simulink model "AcasXuClosedLoop_m_1"  (R2019b)
settings: Solver=VariableStepAuto  StartTime=0.0  StopTime=30  RelTol=1e-3
libraries: neural x1560, simulink x2
(part 4 of 85)

== system AcasXuClosedLoop_m_1/networks/AcasXu_4_1/Layer 3 ==
  "a{2} " : Inport  PortDimensions=50
      mask Display: e = 0.06;c1 = [120 230 180]/255;c2 = ([120 230 180]+0)/(256+128);c3 = ([120 230 180]+128)/(256+128);patch([0 1 1 0],[0 0 1 1],c1);patch([0 1 1 1-e 1-e 0+e],[0 0 1 1-e 0+e 0+e],c2);patch([0 0 1 1-e 0+e 0+e],[0 1 1 1-e 1-e 0+e],c3);plot([0 1 1 0 0],[0 0 1 1 0]);
  Delays 1 : Subsystem
      mask Display: e = 0.06;c1 = [120 150 230]/255;c2 = ([120 150 230]+0)/383;c3 = ([120 150 230]+128)/383;patch([0 1 1 0],[0 0 1 1],c1);patch([0 1 1 1-e 1-e 0+e],[0 0 1 1-e 0+e 0+e],c2);patch([0 0 1 1-e 0+e 0+e],[0 1 1 1-e 1-e 0+e],c3);plot([0 1 1 0 0],[0 0 1 1 0]);disp('0');
  "LW{3,2}" : Subsystem
      mask Display: e = 0.06;c1 = [120 150 230]/255;c2 = ([120 150 230]+0)/383;c3 = ([120 150 230]+128)/383;patch([0 1 1 0],[0 0 1 1],c1);patch([0 1 1 1-e 1-e 0+e],[0 0 1 1-e 0+e 0+e],c2);patch([0 0 1 1-e 0+e 0+e],[0 1 1 1-e 1-e 0+e],c3);plot([0 1 1 0 0],[0 0 1 1 0]);disp('W');
  "b{3}" : Constant  Value=[0.75966199999999994840749195645912550389766693115234375;-0.838961999999999985533349899924360215663909912109375;-1.1200300000000000810729261502274312078952789306640625;-0.51097300000000001052313791660708375275135040283203125;-0.135124999999999995115018691649311222136020660400390625;-0.82995099999999999429434183184639550745487213134765625;-0.7141610000000000457731630376656539738178253173828125;1.510499999999999953814722175593487918376922607421875;0.282934999999999992059684927880880422890186309814453125;-0.294370999999999993779198348420322872698307037353515625;-0.455872999999999972686737237381748855113983154296875;-0.7350980000000000291748847303097136318683624267578125;-0.36855599999999999472066747330245561897754669189453125;-0.141824000000000005616840326183591969311237335205078125;-0.9845960000000000267306177192949689924716949462890625;-0.1444709999999999883169010672645526938140392303466796875;0.63247799999999998465938233493943698704242706298828125;-0.6318770000000000219841922444174997508525848388671875;-0.00854197999999999936504568864847897202707827091217041015625;0.61706099999999997063326873103505931794643402099609375;-1.305309999999999970299313645227812230587005615234375;0.65445100000000000495248286824789829552173614501953125;-0.8968920000000000225526264330255798995494842529296875;0.022811299999999999632560587770058191381394863128662109375;-0.347494000000000025085711286010337062180042266845703125;-0.138658000000000003471001264188089407980442047119140625;-0.81998499999999996390442902338691055774688720703125;-1.0180700000000000304822833641082979738712310791015625;-0.88269600000000003614530896811629645526409149169921875;-1.585620000000000029416469260468147695064544677734375;-1.1131299999999999528199623455293476581573486328125;-0.888298999999999949750417727045714855194091796875;-1.0311099999999999710098563809879124164581298828125;-0.48253800000000002246025587737676687538623809814453125;-0.363474000000000019294787989565520547330379486083984375;-0.670150000000000023447910280083306133747100830078125;-0.645361999999999991217691786005161702632904052734375;0.36204300000000000370192765331012196838855743408203125;-1.3692699999999999871391764827421866357326507568359375;-2.15331999999999990080823408789001405239105224609375;0.321091999999999988535392958510783500969409942626953125;1.4917700000000000404298816647497005760669708251953125;0.1303020000000000011564083024495630525052547454833984375;-0.7060370000000000256790144703700207173824310302734375;1.1547400000000000996891458271420560777187347412109375;-0.73546699999999998187405481075984425842761993408203125;-0.207056999999999991057819670459139160811901092529296875;-0.95738800000000001677591399129596538841724395751953125;-1.3000700000000000589039927945123054087162017822265625;-0.1655649999999999899547020731915836222469806671142578125]
      mask Display: e = 0.06;c1 = [120 150 230]/255;c2 = ([120 150 230]+0)/383;c3 = ([120 150 230]+128)/383;patch([0 1 1 0],[0 0 1 1],c1);patch([0 1 1 1-e 1-e 0+e],[0 0 1 1-e 0+e 0+e],c2);patch([0 0 1 1-e 0+e 0+e],[0 1 1 1-e 1-e 0+e],c3);plot([0 1 1 0 0],[0 0 1 1 0]);disp('b');
  netsum : Sum  Inputs=2  SaturateOnIntegerOverflow=on  InputSameDT=on  OutDataTypeStr=Inherit: Same as first input
      mask Display: e = 0.06;c1 = [120 150 230]/255;c2 = ([120 150 230]+0)/383;c3 = ([120 150 230]+128)/383;patch([0 1 1 0],[0 0 1 1],c1);patch([0 1 1 1-e 1-e 0+e],[0 0 1 1-e 0+e 0+e],c2);patch([0 0 1 1-e 0+e 0+e],[0 1 1 1-e 1-e 0+e],c3);plot([0 1 1 0 0],[0 0 1 1 0]);disp('+');
  tansig : neural/Transfer Functions/tansig
      settings: SourceProductName=Deep Learning Toolbox
  "a{3}" : Outport  InitialOutput=[0;0;0;0;0;0;0;0;0;0;0;0;0;0;0;0;0;0;0;0;0;0;0;0;0;0;0;0;0;0;0;0;0;0;0;0;0;0;0;0;0;0;0;0;0;0;0;0;0;0]
      mask Display: e = 0.06;c1 = [120 230 180]/255;c2 = ([120 230 180]+0)/(256+128);c3 = ([120 230 180]+128)/(256+128);patch([0 1 1 0],[0 0 1 1],c1);patch([0 1 1 1-e 1-e 0+e],[0 0 1 1-e 0+e 0+e],c2);patch([0 0 1 1-e 0+e 0+e],[0 1 1 1-e 1-e 0+e],c3);plot([0 1 1 0 0],[0 0 1 1 0]);
  wires:
  tansig/1 -> "a{3}"/1
  netsum/1 -> tansig/1
  "b{3}"/1 -> netsum/2
  "LW{3,2}"/1("lz{3,2}") -> netsum/1
  Delays 1/1("pd{3,2}") -> "LW{3,2}"/1("ad{3,2}")
  "a{2} "/1 -> Delays 1/1("p{3}")

== system AcasXuClosedLoop_m_1/networks/AcasXu_4_1/Layer 4 ==
  "a{3} " : Inport  PortDimensions=50
      mask Display: e = 0.06;c1 = [120 230 180]/255;c2 = ([120 230 180]+0)/(256+128);c3 = ([120 230 180]+128)/(256+128);patch([0 1 1 0],[0 0 1 1],c1);patch([0 1 1 1-e 1-e 0+e],[0 0 1 1-e 0+e 0+e],c2);patch([0 0 1 1-e 0+e 0+e],[0 1 1 1-e 1-e 0+e],c3);plot([0 1 1 0 0],[0 0 1 1 0]);
  Delays 1 : Subsystem
      mask Display: e = 0.06;c1 = [120 150 230]/255;c2 = ([120 150 230]+0)/383;c3 = ([120 150 230]+128)/383;patch([0 1 1 0],[0 0 1 1],c1);patch([0 1 1 1-e 1-e 0+e],[0 0 1 1-e 0+e 0+e],c2);patch([0 0 1 1-e 0+e 0+e],[0 1 1 1-e 1-e 0+e],c3);plot([0 1 1 0 0],[0 0 1 1 0]);disp('0');
  "LW{4,3}" : Subsystem
      mask Display: e = 0.06;c1 = [120 150 230]/255;c2 = ([120 150 230]+0)/383;c3 = ([120 150 230]+128)/383;patch([0 1 1 0],[0 0 1 1],c1);patch([0 1 1 1-e 1-e 0+e],[0 0 1 1-e 0+e 0+e],c2);patch([0 0 1 1-e 0+e 0+e],[0 1 1 1-e 1-e 0+e],c3);plot([0 1 1 0 0],[0 0 1 1 0]);disp('W');
  "b{4}" : Constant  Value=[-0.6820079999999999476045786650502122938632965087890625;-3.08436999999999983401721692644059658050537109375;0.585555999999999965410779623198322951793670654296875;-0.5398359999999999825348595550167374312877655029296875;-0.55025299999999999212008106042048893868923187255859375;0.0256048000000000004761080418802521307952702045440673828125;-1.7290099999999999358379909608629532158374786376953125;-0.1298610000000000042064129956997931003570556640625;-0.8305789999999999562163566224626265466213226318359375;-0.196811999999999986954435371444560587406158447265625;-0.6160639999999999449897813974530436098575592041015625;0.3433990000000000097912788987741805613040924072265625;-1.597210000000000018616219676914624869823455810546875;0.1576450000000000073452355309200356714427471160888671875;0.88317800000000001858779796748422086238861083984375;-0.70011999999999996457944462235900573432445526123046875;-0.286934000000000022367885321727953851222991943359375;0.637162000000000006139089236967265605926513671875;1.2516700000000000603250782660325057804584503173828125;-0.01162849999999999994759747323769261129200458526611328125;-0.5578469999999999817674734003958292305469512939453125;-1.00337999999999993860910763032734394073486328125;1.05571999999999999175770426518283784389495849609375;-1.24138999999999999346300683100707828998565673828125;0.186377999999999988123278171769925393164157867431640625;0.0017374199999999999366462333227900671772658824920654296875;0.105161000000000004472866521609830670058727264404296875;0.54805800000000004512656914812396280467510223388671875;0.08856619999999999770512459917881642468273639678955078125;0.1579730000000000023074875343809253536164760589599609375;-0.0757977999999999985103471544789499603211879730224609375;1.2585900000000000975575176198617555201053619384765625;-1.461959999999999926245664028101600706577301025390625;0.62902299999999999879918277656543068587779998779296875;-0.7479839999999999822222207512822933495044708251953125;0.09964230000000000309068326487249578349292278289794921875;1.006110000000000059827698351000435650348663330078125;0.77711699999999994670218939063488505780696868896484375;0.325390000000000012558842854559770785272121429443359375;-1.7636499999999999399591388282715342938899993896484375;-0.53327899999999994751220810940139926970005035400390625;-0.77692799999999995197441648997482843697071075439453125;-0.73104299999999999837285713510937057435512542724609375;0.64756599999999997496757941917167045176029205322265625;-0.1434709999999999874287226475644274614751338958740234375;0.751273999999999997356781022972427308559417724609375;0.4473059999999999813979911778005771338939666748046875;1.2945800000000000640199004919850267469882965087890625;-0.55212600000000000566302560400799848139286041259765625;1.038089999999999957225327307241968810558319091796875]
      mask Display: e = 0.06;c1 = [120 150 230]/255;c2 = ([120 150 230]+0)/383;c3 = ([120 150 230]+128)/383;patch([0 1 1 0],[0 0 1 1],c1);patch([0 1 1 1-e 1-e 0+e],[0 0 1 1-e 0+e 0+e],c2);patch([0 0 1 1-e 0+e 0+e],[0 1 1 1-e 1-e 0+e],c3);plot([0 1 1 0 0],[0 0 1 1 0]);disp('b');
  netsum : Sum  Inputs=2  SaturateOnIntegerOverflow=on  InputSameDT=on  OutDataTypeStr=Inherit: Same as first input
      mask Display: e = 0.06;c1 = [120 150 230]/255;c2 = ([120 150 230]+0)/383;c3 = ([120 150 230]+128)/383;patch([0 1 1 0],[0 0 1 1],c1);patch([0 1 1 1-e 1-e 0+e],[0 0 1 1-e 0+e 0+e],c2);patch([0 0 1 1-e 0+e 0+e],[0 1 1 1-e 1-e 0+e],c3);plot([0 1 1 0 0],[0 0 1 1 0]);disp('+');
  tansig : neural/Transfer Functions/tansig
      settings: SourceProductName=Deep Learning Toolbox
  "a{4}" : Outport  InitialOutput=[0;0;0;0;0;0;0;0;0;0;0;0;0;0;0;0;0;0;0;0;0;0;0;0;0;0;0;0;0;0;0;0;0;0;0;0;0;0;0;0;0;0;0;0;0;0;0;0;0;0]
      mask Display: e = 0.06;c1 = [120 230 180]/255;c2 = ([120 230 180]+0)/(256+128);c3 = ([120 230 180]+128)/(256+128);patch([0 1 1 0],[0 0 1 1],c1);patch([0 1 1 1-e 1-e 0+e],[0 0 1 1-e 0+e 0+e],c2);patch([0 0 1 1-e 0+e 0+e],[0 1 1 1-e 1-e 0+e],c3);plot([0 1 1 0 0],[0 0 1 1 0]);
  wires:
  tansig/1 -> "a{4}"/1
  netsum/1 -> tansig/1
  "b{4}"/1 -> netsum/2
  "LW{4,3}"/1("lz{4,3}") -> netsum/1
  Delays 1/1("pd{4,3}") -> "LW{4,3}"/1("ad{4,3}")
  "a{3} "/1 -> Delays 1/1("p{4}")

== system AcasXuClosedLoop_m_1/networks/AcasXu_4_1/Layer 5 ==
  "a{4} " : Inport  PortDimensions=50
      mask Display: e = 0.06;c1 = [120 230 180]/255;c2 = ([120 230 180]+0)/(256+128);c3 = ([120 230 180]+128)/(256+128);patch([0 1 1 0],[0 0 1 1],c1);patch([0 1 1 1-e 1-e 0+e],[0 0 1 1-e 0+e 0+e],c2);patch([0 0 1 1-e 0+e 0+e],[0 1 1 1-e 1-e 0+e],c3);plot([0 1 1 0 0],[0 0 1 1 0]);
  Delays 1 : Subsystem
      mask Display: e = 0.06;c1 = [120 150 230]/255;c2 = ([120 150 230]+0)/383;c3 = ([120 150 230]+128)/383;patch([0 1 1 0],[0 0 1 1],c1);patch([0 1 1 1-e 1-e 0+e],[0 0 1 1-e 0+e 0+e],c2);patch([0 0 1 1-e 0+e 0+e],[0 1 1 1-e 1-e 0+e],c3);plot([0 1 1 0 0],[0 0 1 1 0]);disp('0');
  "LW{5,4}" : Subsystem
      mask Display: e = 0.06;c1 = [120 150 230]/255;c2 = ([120 150 230]+0)/383;c3 = ([120 150 230]+128)/383;patch([0 1 1 0],[0 0 1 1],c1);patch([0 1 1 1-e 1-e 0+e],[0 0 1 1-e 0+e 0+e],c2);patch([0 0 1 1-e 0+e 0+e],[0 1 1 1-e 1-e 0+e],c3);plot([0 1 1 0 0],[0 0 1 1 0]);disp('W');
  "b{5}" : Constant  Value=[-1.148800000000000043343106881366111338138580322265625;-1.268780000000000018900436771218664944171905517578125;-0.448139999999999982804865794605575501918792724609375;0.4046790000000000109281472759903408586978912353515625;1.01714999999999999857891452847979962825775146484375;0.305279000000000022563284574061981402337551116943359375;0.08392149999999999610000855909675010479986667633056640625;0.52215100000000003177547114319168031215667724609375;-1.074980000000000046611603465862572193145751953125;-1.4273800000000000931521526581491343677043914794921875;0.52887099999999998001243284306838177144527435302734375;-0.284766999999999992354560163221322000026702880859375;0.462851999999999985657694878682377748191356658935546875;-1.434930000000000038795633372501470148563385009765625;1.021269999999999900097691352129913866519927978515625;1.4297100000000000363797880709171295166015625;-0.55277399999999998758681840627104975283145904541015625;-1.43315999999999998948396751075051724910736083984375;0.64438099999999998157562686174060218036174774169921875;1.3235900000000000442668124378542415797710418701171875;-0.356341000000000018843593352357856929302215576171875;-1.3253399999999999625543978254427202045917510986328125;0.47899700000000000610356210017926059663295745849609375;0.09044280000000000374615893861118820495903491973876953125;-0.1897939999999999904911618386904592625796794891357421875;0.081688700000000002976463520099059678614139556884765625;-0.1393810000000000048903103788688895292580127716064453125;0.79328699999999996439470351106137968599796295166015625;0.853005000000000013216094885137863457202911376953125;0.8116689999999999738378164693131111562252044677734375;0.1342210000000000069686478809671825729310512542724609375;-0.89552500000000001545430450278217904269695281982421875;0.41882399999999997408650642682914622128009796142578125;0.5555499999999999882760448599583469331264495849609375;0.2302760000000000084607876260633929632604122161865234375;1.2937499999999999555910790149937383830547332763671875;0.65880199999999999871391764827421866357326507568359375;0.387861999999999984556353638254222460091114044189453125;-0.1655999999999999972022379779446055181324481964111328125;1.0075700000000000766675611885148100554943084716796875;0.194539999999999990709653729936690069735050201416015625;-1.03254000000000001335820343228988349437713623046875;-0.144120999999999999108268866621074266731739044189453125;0.42739700000000002688693712116219103336334228515625;-1.1556599999999999095479097377392463386058807373046875;1.261789999999999967172925607883371412754058837890625;-0.282252000000000002888356220864807255566120147705078125;-0.00985550999999999961798113901068063569255173206329345703125;0.88892300000000001869437937784823589026927947998046875;2.444459999999999855191390452091582119464874267578125]
      mask Display: e = 0.06;c1 = [120 150 230]/255;c2 = ([120 150 230]+0)/383;c3 = ([120 150 230]+128)/383;patch([0 1 1 0],[0 0 1 1],c1);patch([0 1 1 1-e 1-e 0+e],[0 0 1 1-e 0+e 0+e],c2);patch([0 0 1 1-e 0+e 0+e],[0 1 1 1-e 1-e 0+e],c3);plot([0 1 1 0 0],[0 0 1 1 0]);disp('b');
  netsum : Sum  Inputs=2  SaturateOnIntegerOverflow=on  InputSameDT=on  OutDataTypeStr=Inherit: Same as first input
      mask Display: e = 0.06;c1 = [120 150 230]/255;c2 = ([120 150 230]+0)/383;c3 = ([120 150 230]+128)/383;patch([0 1 1 0],[0 0 1 1],c1);patch([0 1 1 1-e 1-e 0+e],[0 0 1 1-e 0+e 0+e],c2);patch([0 0 1 1-e 0+e 0+e],[0 1 1 1-e 1-e 0+e],c3);plot([0 1 1 0 0],[0 0 1 1 0]);disp('+');
  tansig : neural/Transfer Functions/tansig
      settings: SourceProductName=Deep Learning Toolbox
  "a{5}" : Outport  InitialOutput=[0;0;0;0;0;0;0;0;0;0;0;0;0;0;0;0;0;0;0;0;0;0;0;0;0;0;0;0;0;0;0;0;0;0;0;0;0;0;0;0;0;0;0;0;0;0;0;0;0;0]
      mask Display: e = 0.06;c1 = [120 230 180]/255;c2 = ([120 230 180]+0)/(256+128);c3 = ([120 230 180]+128)/(256+128);patch([0 1 1 0],[0 0 1 1],c1);patch([0 1 1 1-e 1-e 0+e],[0 0 1 1-e 0+e 0+e],c2);patch([0 0 1 1-e 0+e 0+e],[0 1 1 1-e 1-e 0+e],c3);plot([0 1 1 0 0],[0 0 1 1 0]);
  wires:
  tansig/1 -> "a{5}"/1
  netsum/1 -> tansig/1
  "b{5}"/1 -> netsum/2
  "LW{5,4}"/1("lz{5,4}") -> netsum/1
  Delays 1/1("pd{5,4}") -> "LW{5,4}"/1("ad{5,4}")
  "a{4} "/1 -> Delays 1/1("p{5}")

== system AcasXuClosedLoop_m_1/networks/AcasXu_4_1/Layer 6 ==
  "a{5} " : Inport  PortDimensions=50
      mask Display: e = 0.06;c1 = [120 230 180]/255;c2 = ([120 230 180]+0)/(256+128);c3 = ([120 230 180]+128)/(256+128);patch([0 1 1 0],[0 0 1 1],c1);patch([0 1 1 1-e 1-e 0+e],[0 0 1 1-e 0+e 0+e],c2);patch([0 0 1 1-e 0+e 0+e],[0 1 1 1-e 1-e 0+e],c3);plot([0 1 1 0 0],[0 0 1 1 0]);
  Delays 1 : Subsystem
      mask Display: e = 0.06;c1 = [120 150 230]/255;c2 = ([120 150 230]+0)/383;c3 = ([120 150 230]+128)/383;patch([0 1 1 0],[0 0 1 1],c1);patch([0 1 1 1-e 1-e 0+e],[0 0 1 1-e 0+e 0+e],c2);patch([0 0 1 1-e 0+e 0+e],[0 1 1 1-e 1-e 0+e],c3);plot([0 1 1 0 0],[0 0 1 1 0]);disp('0');
  "LW{6,5}" : Subsystem
      mask Display: e = 0.06;c1 = [120 150 230]/255;c2 = ([120 150 230]+0)/383;c3 = ([120 150 230]+128)/383;patch([0 1 1 0],[0 0 1 1],c1);patch([0 1 1 1-e 1-e 0+e],[0 0 1 1-e 0+e 0+e],c2);patch([0 0 1 1-e 0+e 0+e],[0 1 1 1-e 1-e 0+e],c3);plot([0 1 1 0 0],[0 0 1 1 0]);disp('W');
  "b{6}" : Constant  Value=[-2.6473800000000000665068000671453773975372314453125;-0.10213899999999999368416325751240947283804416656494140625;0.09831600000000000061373128801278653554618358612060546875;0.2058689999999999964419572506812983192503452301025390625;-0.0282583999999999994912069922747832606546580791473388671875;0.196272000000000002017941369558684527873992919921875;-0.4957759999999999944719775157864205539226531982421875;-0.031972300000000002107025665054607088677585124969482421875;0.03432000000000000328181926079196273349225521087646484375;-0.005902010000000000068676175857262933277525007724761962890625;-0.08618030000000000134807720542085007764399051666259765625;-0.08027869999999999450768228825836558826267719268798828125;0.1025480000000000002646771690706373192369937896728515625;-0.09591170000000000250839349291709368117153644561767578125;-1.2270700000000001050892706189188174903392791748046875;0.14760200000000001097077984013594686985015869140625;-0.00941825999999999947942530553746109944768249988555908203125;-0.8689810000000000034248159863636828958988189697265625;-0.419634000000000007002398660915787331759929656982421875;-1.061059999999999892139612711616791784763336181640625;-0.234507999999999994233945699306786991655826568603515625;0.57218599999999997240962557043530978262424468994140625;0.3316470000000000251105802817619405686855316162109375;-1.96290999999999993264054864994250237941741943359375;-0.4404660000000000241726638705586083233356475830078125;-0.20329900000000000748201500755385495722293853759765625;-0.132805000000000006377121053446899168193340301513671875;-0.03263760000000000272013522817360353656113147735595703125;-0.472158000000000022122748077890719287097454071044921875;-0.54876899999999995127808460892993025481700897216796875;-1.289099999999999912603243501507677137851715087890625;0.037761700000000002208633276268301415257155895233154296875;0.2109080000000000121307408562643104232847690582275390625;0.41221600000000002683719912965898402035236358642578125;0.1534149999999999958166796432124101556837558746337890625;-0.598470999999999975216269376687705516815185546875;-0.5960170000000000189999127542250789701938629150390625;-2.02934999999999998721023075631819665431976318359375;0.36855599999999999472066747330245561897754669189453125;0.176721999999999990205168387547018937766551971435546875;-0.72194700000000000539301936441916041076183319091796875;0.30531099999999999905497816143906675279140472412109375;0.3467620000000000146656020660884678363800048828125;-0.09170309999999999572839470829421770758926868438720703125;-2.207030000000000047322146201622672379016876220703125;-0.932763000000000008782308213994838297367095947265625;-0.377265000000000016999734953060396946966648101806640625;-1.375010000000000065512040237081237137317657470703125;-1.0118899999999999561595132036018185317516326904296875;0.2037650000000000016786572132332366891205310821533203125]
      mask Display: e = 0.06;c1 = [120 150 230]/255;c2 = ([120 150 230]+0)/383;c3 = ([120 150 230]+128)/383;patch([0 1 1 0],[0 0 1 1],c1);patch([0 1 1 1-e 1-e 0+e],[0 0 1 1-e 0+e 0+e],c2);patch([0 0 1 1-e 0+e 0+e],[0 1 1 1-e 1-e 0+e],c3);plot([0 1 1 0 0],[0 0 1 1 0]);disp('b');
  netsum : Sum  Inputs=2  SaturateOnIntegerOverflow=on  InputSameDT=on  OutDataTypeStr=Inherit: Same as first input
      mask Display: e = 0.06;c1 = [120 150 230]/255;c2 = ([120 150 230]+0)/383;c3 = ([120 150 230]+128)/383;patch([0 1 1 0],[0 0 1 1],c1);patch([0 1 1 1-e 1-e 0+e],[0 0 1 1-e 0+e 0+e],c2);patch([0 0 1 1-e 0+e 0+e],[0 1 1 1-e 1-e 0+e],c3);plot([0 1 1 0 0],[0 0 1 1 0]);disp('+');
  tansig : neural/Transfer Functions/tansig
      settings: SourceProductName=Deep Learning Toolbox
  "a{6}" : Outport  InitialOutput=[0;0;0;0;0;0;0;0;0;0;0;0;0;0;0;0;0;0;0;0;0;0;0;0;0;0;0;0;0;0;0;0;0;0;0;0;0;0;0;0;0;0;0;0;0;0;0;0;0;0]
      mask Display: e = 0.06;c1 = [120 230 180]/255;c2 = ([120 230 180]+0)/(256+128);c3 = ([120 230 180]+128)/(256+128);patch([0 1 1 0],[0 0 1 1],c1);patch([0 1 1 1-e 1-e 0+e],[0 0 1 1-e 0+e 0+e],c2);patch([0 0 1 1-e 0+e 0+e],[0 1 1 1-e 1-e 0+e],c3);plot([0 1 1 0 0],[0 0 1 1 0]);
  wires:
  tansig/1 -> "a{6}"/1
  netsum/1 -> tansig/1
  "b{6}"/1 -> netsum/2
  "LW{6,5}"/1("lz{6,5}") -> netsum/1
  Delays 1/1("pd{6,5}") -> "LW{6,5}"/1("ad{6,5}")
  "a{5} "/1 -> Delays 1/1("p{6}")

== system AcasXuClosedLoop_m_1/networks/AcasXu_4_1/Layer 7 ==
  "a{6} " : Inport  PortDimensions=50
      mask Display: e = 0.06;c1 = [120 230 180]/255;c2 = ([120 230 180]+0)/(256+128);c3 = ([120 230 180]+128)/(256+128);patch([0 1 1 0],[0 0 1 1],c1);patch([0 1 1 1-e 1-e 0+e],[0 0 1 1-e 0+e 0+e],c2);patch([0 0 1 1-e 0+e 0+e],[0 1 1 1-e 1-e 0+e],c3);plot([0 1 1 0 0],[0 0 1 1 0]);
  Delays 1 : Subsystem
      mask Display: e = 0.06;c1 = [120 150 230]/255;c2 = ([120 150 230]+0)/383;c3 = ([120 150 230]+128)/383;patch([0 1 1 0],[0 0 1 1],c1);patch([0 1 1 1-e 1-e 0+e],[0 0 1 1-e 0+e 0+e],c2);patch([0 0 1 1-e 0+e 0+e],[0 1 1 1-e 1-e 0+e],c3);plot([0 1 1 0 0],[0 0 1 1 0]);disp('0');
  "LW{7,6}" : Subsystem
      mask Display: e = 0.06;c1 = [120 150 230]/255;c2 = ([120 150 230]+0)/383;c3 = ([120 150 230]+128)/383;patch([0 1 1 0],[0 0 1 1],c1);patch([0 1 1 1-e 1-e 0+e],[0 0 1 1-e 0+e 0+e],c2);patch([0 0 1 1-e 0+e 0+e],[0 1 1 1-e 1-e 0+e],c3);plot([0 1 1 0 0],[0 0 1 1 0]);disp('W');
  "b{7}" : Constant  Value=[-0.020869800000000000850253201178929884918034076690673828125;-0.01825859999999999983000265046939603053033351898193359375;0.0181765000000000016833201499366623465903103351593017578125;-0.018426800000000000123723253864227444864809513092041015625;0.01793809999999999849062959356160718016326427459716796875]
      mask Display: e = 0.06;c1 = [120 150 230]/255;c2 = ([120 150 230]+0)/383;c3 = ([120 150 230]+128)/383;patch([0 1 1 0],[0 0 1 1],c1);patch([0 1 1 1-e 1-e 0+e],[0 0 1 1-e 0+e 0+e],c2);patch([0 0 1 1-e 0+e 0+e],[0 1 1 1-e 1-e 0+e],c3);plot([0 1 1 0 0],[0 0 1 1 0]);disp('b');
  netsum : Sum  Inputs=2  SaturateOnIntegerOverflow=on  InputSameDT=on  OutDataTypeStr=Inherit: Same as first input
      mask Display: e = 0.06;c1 = [120 150 230]/255;c2 = ([120 150 230]+0)/383;c3 = ([120 150 230]+128)/383;patch([0 1 1 0],[0 0 1 1],c1);patch([0 1 1 1-e 1-e 0+e],[0 0 1 1-e 0+e 0+e],c2);patch([0 0 1 1-e 0+e 0+e],[0 1 1 1-e 1-e 0+e],c3);plot([0 1 1 0 0],[0 0 1 1 0]);disp('+');
  purelin : neural/Transfer Functions/purelin
      settings: SourceProductName=Deep Learning Toolbox
  "a{7}" : Outport  InitialOutput=[0;0;0;0;0]
      mask Display: e = 0.06;c1 = [120 230 180]/255;c2 = ([120 230 180]+0)/(256+128);c3 = ([120 230 180]+128)/(256+128);patch([0 1 1 0],[0 0 1 1],c1);patch([0 1 1 1-e 1-e 0+e],[0 0 1 1-e 0+e 0+e],c2);patch([0 0 1 1-e 0+e 0+e],[0 1 1 1-e 1-e 0+e],c3);plot([0 1 1 0 0],[0 0 1 1 0]);
  wires:
  purelin/1 -> "a{7}"/1
  netsum/1 -> purelin/1
  "b{7}"/1 -> netsum/2
  "LW{7,6}"/1("lz{7,6}") -> netsum/1
  Delays 1/1("pd{7,6}") -> "LW{7,6}"/1("ad{7,6}")
  "a{6} "/1 -> Delays 1/1("p{7}")

== system AcasXuClosedLoop_m_1/networks/AcasXu_4_1/Process Input 1 ==
  x : Inport  PortDimensions=5
      mask Display: e = 0.06;c1 = [120 230 180]/255;c2 = ([120 230 180]+0)/(256+128);c3 = ([120 230 180]+128)/(256+128);patch([0 1 1 0],[0 0 1 1],c1);patch([0 1 1 1-e 1-e 0+e],[0 0 1 1-e 0+e 0+e],c2);patch([0 0 1 1-e 0+e 0+e],[0 1 1 1-e 1-e 0+e],c3);plot([0 1 1 0 0],[0 0 1 1 0]);
  p : Outport  PortDimensions=5
      mask Display: e = 0.06;c1 = [120 230 180]/255;c2 = ([120 230 180]+0)/(256+128);c3 = ([120 230 180]+128)/(256+128);patch([0 1 1 0],[0 0 1 1],c1);patch([0 1 1 1-e 1-e 0+e],[0 0 1 1-e 0+e 0+e],c2);patch([0 0 1 1-e 0+e 0+e],[0 1 1 1-e 1-e 0+e],c3);plot([0 1 1 0 0],[0 0 1 1 0]);
  wires:
  x/1 -> p/1

== system AcasXuClosedLoop_m_1/networks/AcasXu_4_1/Process Output 1 ==
  a : Inport  PortDimensions=5
      mask Display: e = 0.06;c1 = [120 230 180]/255;c2 = ([120 230 180]+0)/(256+128);c3 = ([120 230 180]+128)/(256+128);patch([0 1 1 0],[0 0 1 1],c1);patch([0 1 1 1-e 1-e 0+e],[0 0 1 1-e 0+e 0+e],c2);patch([0 0 1 1-e 0+e 0+e],[0 1 1 1-e 1-e 0+e],c3);plot([0 1 1 0 0],[0 0 1 1 0]);
  y : Outport  PortDimensions=5
      mask Display: e = 0.06;c1 = [120 230 180]/255;c2 = ([120 230 180]+0)/(256+128);c3 = ([120 230 180]+128)/(256+128);patch([0 1 1 0],[0 0 1 1],c1);patch([0 1 1 1-e 1-e 0+e],[0 0 1 1-e 0+e 0+e],c2);patch([0 0 1 1-e 0+e 0+e],[0 1 1 1-e 1-e 0+e],c3);plot([0 1 1 0 0],[0 0 1 1 0]);
  wires:
  a/1 -> y/1

== system AcasXuClosedLoop_m_1/networks/AcasXu_5_1/Layer 1 ==
  "p{1}" : Inport  PortDimensions=5
      mask Display: e = 0.06;c1 = [120 230 180]/255;c2 = ([120 230 180]+0)/(256+128);c3 = ([120 230 180]+128)/(256+128);patch([0 1 1 0],[0 0 1 1],c1);patch([0 1 1 1-e 1-e 0+e],[0 0 1 1-e 0+e 0+e],c2);patch([0 0 1 1-e 0+e 0+e],[0 1 1 1-e 1-e 0+e],c3);plot([0 1 1 0 0],[0 0 1 1 0]);
  Delays 1 : Subsystem
      mask Display: e = 0.06;c1 = [120 150 230]/255;c2 = ([120 150 230]+0)/383;c3 = ([120 150 230]+128)/383;patch([0 1 1 0],[0 0 1 1],c1);patch([0 1 1 1-e 1-e 0+e],[0 0 1 1-e 0+e 0+e],c2);patch([0 0 1 1-e 0+e 0+e],[0 1 1 1-e 1-e 0+e],c3);plot([0 1 1 0 0],[0 0 1 1 0]);disp('0');
  "IW{1,1}" : Subsystem
      mask Display: e = 0.06;c1 = [120 150 230]/255;c2 = ([120 150 230]+0)/383;c3 = ([120 150 230]+128)/383;patch([0 1 1 0],[0 0 1 1],c1);patch([0 1 1 1-e 1-e 0+e],[0 0 1 1-e 0+e 0+e],c2);patch([0 0 1 1-e 0+e 0+e],[0 1 1 1-e 1-e 0+e],c3);plot([0 1 1 0 0],[0 0 1 1 0]);disp('W');
  "b{1}" : Constant  Value=[0.27264399999999999746336243333644233644008636474609375;-0.7264909999999999978825826474349014461040496826171875;-0.77816899999999999959499064061674289405345916748046875;0.2486210000000000086561868783974205143749713897705078125;0.1726000000000000034194869158454821445047855377197265625;0.031532100000000000405986355644927243702113628387451171875;-0.084186499999999997445598864942439831793308258056640625;0.070256299999999993755039895404479466378688812255859375;-0.264100999999999974665598756473627872765064239501953125;-0.005442909999999999588748966772300263983197510242462158203125;0.282386999999999999122479721336276270449161529541015625;-0.6244279999999999830606611794792115688323974609375;-0.6145469999999999544115780736319720745086669921875;-0.0305731999999999982942089360449244850315153598785400390625;0.251867000000000007542411140093463473021984100341796875;-0.719573000000000018161472326028160750865936279296875;-0.408038999999999985046628125928691588342189788818359375;0.19076999999999999513278226004331372678279876708984375;-0.458693999999999990624388601645478047430515289306640625;0.11665899999999999880895273918213206343352794647216796875;0.021026099999999998957367353114022989757359027862548828125;-0.2186200000000000087663210024402360431849956512451171875;0.039987099999999997645971916426788084208965301513671875;-0.7091380000000000460858018414000980556011199951171875;-0.08869570000000000231654695426186663098633289337158203125;0.01514509999999999988185006571939084096811711788177490234375;-0.5971290000000000208757455766317434608936309814453125;-0.373078999999999993963939459717948921024799346923828125;-0.2486629999999999951487694715979159809648990631103515625;-0.45685100000000000708411107552819885313510894775390625;-0.0294940999999999987901677656054744147695600986480712890625;-0.5039919999999999955520024741417728364467620849609375;-0.450427999999999995051069845430902205407619476318359375;-0.383678000000000019031887177334283478558063507080078125;-0.00826648999999999960219820849260941031388938426971435546875;0.52696200000000004148859034103224985301494598388671875;-0.54082600000000002893330020015127956867218017578125;-0.0591807000000000027473134878164273686707019805908203125;-0.257616000000000011649348152786842547357082366943359375;-0.0716877999999999959701568741365917958319187164306640625;-0.7003369999999999873097067393246106803417205810546875;-0.176420999999999994489741084180423058569431304931640625;-0.348355000000000025739410602909629233181476593017578125;0.26371299999999997520916394933010451495647430419921875;-0.0024396199999999999830091468311366043053567409515380859375;0.10330999999999999905408998301936662755906581878662109375;0.0286719000000000001637801005927030928432941436767578125;-0.53494900000000000783728637543390505015850067138671875;-0.0248139999999999992519317260075695230625569820404052734375;0.440342999999999984428455945817404426634311676025390625]
      mask Display: e = 0.06;c1 = [120 150 230]/255;c2 = ([120 150 230]+0)/383;c3 = ([120 150 230]+128)/383;patch([0 1 1 0],[0 0 1 1],c1);patch([0 1 1 1-e 1-e 0+e],[0 0 1 1-e 0+e 0+e],c2);patch([0 0 1 1-e 0+e 0+e],[0 1 1 1-e 1-e 0+e],c3);plot([0 1 1 0 0],[0 0 1 1 0]);disp('b');
  netsum : Sum  Inputs=2  SaturateOnIntegerOverflow=on  InputSameDT=on  OutDataTypeStr=Inherit: Same as first input
      mask Display: e = 0.06;c1 = [120 150 230]/255;c2 = ([120 150 230]+0)/383;c3 = ([120 150 230]+128)/383;patch([0 1 1 0],[0 0 1 1],c1);patch([0 1 1 1-e 1-e 0+e],[0 0 1 1-e 0+e 0+e],c2);patch([0 0 1 1-e 0+e 0+e],[0 1 1 1-e 1-e 0+e],c3);plot([0 1 1 0 0],[0 0 1 1 0]);disp('+');
  tansig : neural/Transfer Functions/tansig
      settings: SourceProductName=Deep Learning Toolbox
  "a{1}" : Outport  InitialOutput=[0;0;0;0;0;0;0;0;0;0;0;0;0;0;0;0;0;0;0;0;0;0;0;0;0;0;0;0;0;0;0;0;0;0;0;0;0;0;0;0;0;0;0;0;0;0;0;0;0;0]
      mask Display: e = 0.06;c1 = [120 230 180]/255;c2 = ([120 230 180]+0)/(256+128);c3 = ([120 230 180]+128)/(256+128);patch([0 1 1 0],[0 0 1 1],c1);patch([0 1 1 1-e 1-e 0+e],[0 0 1 1-e 0+e 0+e],c2);patch([0 0 1 1-e 0+e 0+e],[0 1 1 1-e 1-e 0+e],c3);plot([0 1 1 0 0],[0 0 1 1 0]);
  wires:
  tansig/1 -> "a{1}"/1
  netsum/1 -> tansig/1
  "b{1}"/1 -> netsum/2
  "IW{1,1}"/1("iz{1,1}") -> netsum/1
  Delays 1/1("pd{1,1}") -> "IW{1,1}"/1("pd{1,1}")
  "p{1}"/1 -> Delays 1/1("p{1}")

== system AcasXuClosedLoop_m_1/networks/AcasXu_5_1/Layer 2 ==
  "a{1} " : Inport  PortDimensions=50
      mask Display: e = 0.06;c1 = [120 230 180]/255;c2 = ([120 230 180]+0)/(256+128);c3 = ([120 230 180]+128)/(256+128);patch([0 1 1 0],[0 0 1 1],c1);patch([0 1 1 1-e 1-e 0+e],[0 0 1 1-e 0+e 0+e],c2);patch([0 0 1 1-e 0+e 0+e],[0 1 1 1-e 1-e 0+e],c3);plot([0 1 1 0 0],[0 0 1 1 0]);
  Delays 1 : Subsystem
      mask Display: e = 0.06;c1 = [120 150 230]/255;c2 = ([120 150 230]+0)/383;c3 = ([120 150 230]+128)/383;patch([0 1 1 0],[0 0 1 1],c1);patch([0 1 1 1-e 1-e 0+e],[0 0 1 1-e 0+e 0+e],c2);patch([0 0 1 1-e 0+e 0+e],[0 1 1 1-e 1-e 0+e],c3);plot([0 1 1 0 0],[0 0 1 1 0]);disp('0');
  "LW{2,1}" : Subsystem
      mask Display: e = 0.06;c1 = [120 150 230]/255;c2 = ([120 150 230]+0)/383;c3 = ([120 150 230]+128)/383;patch([0 1 1 0],[0 0 1 1],c1);patch([0 1 1 1-e 1-e 0+e],[0 0 1 1-e 0+e 0+e],c2);patch([0 0 1 1-e 0+e 0+e],[0 1 1 1-e 1-e 0+e],c3);plot([0 1 1 0 0],[0 0 1 1 0]);disp('W');
  "b{2}" : Constant  Value=[0.69435400000000002673772314665256999433040618896484375;-0.208757999999999999118927007657475769519805908203125;-0.3371049999999999879918277656543068587779998779296875;0.395558000000000020701662606370518915355205535888671875;-1.0438400000000001011102312986622564494609832763671875;0.075501600000000002044231450781808234751224517822265625;-1.16669000000000000483169060316868126392364501953125;0.10205999999999999794386695839421008713543415069580078125;-0.2062150000000000094058094646243262104690074920654296875;-0.2491279999999999883453227766949567012488842010498046875;-0.292478999999999988990140309397247619926929473876953125;-1.1702999999999998959054892111453227698802947998046875;-1.280909999999999993036681189551018178462982177734375;-0.77106200000000002514610741854994557797908782958984375;-0.01460879999999999991067145543865990475751459598541259765625;-0.1493609999999999937703165642233216203749179840087890625;-0.76321399999999994800958802443346939980983734130859375;1.0952200000000000823519030745956115424633026123046875;0.2091240000000000043289816176184103824198246002197265625;1.4441100000000000047606363295926712453365325927734375;0.1825569999999999970530240034349844790995121002197265625;0.461874999999999980015985556747182272374629974365234375;-1.1703799999999999759126012577326036989688873291015625;0.6556729999999999503046410609385930001735687255859375;-0.05577669999999999850270882006952888332307338714599609375;-0.489686999999999983401721692644059658050537109375;1.0898399999999999199218336798367090523242950439453125;0.2116010000000000113029585691037937067449092864990234375;0.53763199999999999878497192185022868216037750244140625;-0.01333890000000000075619510653268662281334400177001953125;-1.1640200000000000546407363799517042934894561767578125;-0.414883999999999975027975551711278967559337615966796875;-0.496560999999999974630071619685622863471508026123046875;-0.0183939000000000012213785538506272132508456707000732421875;0.2301870000000000027196023211217834614217281341552734375;-0.1089299999999999990496490909208660013973712921142578125;-0.73875999999999997225330616856808774173259735107421875;0.097548899999999993948307519531226716935634613037109375;0.4301559999999999828190766493207775056362152099609375;-0.014394099999999999950350826338762999512255191802978515625;-0.0091775699999999994782573509155554347671568393707275390625;0.134299000000000001708855279503040947020053863525390625;-0.015574799999999999755573298898525536060333251953125;-0.78898999999999996912691813122364692389965057373046875;-0.146892999999999995797139717979007400572299957275390625;-0.85777300000000000768096697356668300926685333251953125;-1.260520000000000084838802649755962193012237548828125;-0.62323099999999997944399865446030162274837493896484375;-0.480572999999999972420283711471711285412311553955078125;0.85980299999999998394883959917933680117130279541015625]
      mask Display: e = 0.06;c1 = [120 150 230]/255;c2 = ([120 150 230]+0)/383;c3 = ([120 150 230]+128)/383;patch([0 1 1 0],[0 0 1 1],c1);patch([0 1 1 1-e 1-e 0+e],[0 0 1 1-e 0+e 0+e],c2);patch([0 0 1 1-e 0+e 0+e],[0 1 1 1-e 1-e 0+e],c3);plot([0 1 1 0 0],[0 0 1 1 0]);disp('b');
  netsum : Sum  Inputs=2  SaturateOnIntegerOverflow=on  InputSameDT=on  OutDataTypeStr=Inherit: Same as first input
      mask Display: e = 0.06;c1 = [120 150 230]/255;c2 = ([120 150 230]+0)/383;c3 = ([120 150 230]+128)/383;patch([0 1 1 0],[0 0 1 1],c1);patch([0 1 1 1-e 1-e 0+e],[0 0 1 1-e 0+e 0+e],c2);patch([0 0 1 1-e 0+e 0+e],[0 1 1 1-e 1-e 0+e],c3);plot([0 1 1 0 0],[0 0 1 1 0]);disp('+');
  tansig : neural/Transfer Functions/tansig
      settings: SourceProductName=Deep Learning Toolbox
  "a{2}" : Outport  InitialOutput=[0;0;0;0;0;0;0;0;0;0;0;0;0;0;0;0;0;0;0;0;0;0;0;0;0;0;0;0;0;0;0;0;0;0;0;0;0;0;0;0;0;0;0;0;0;0;0;0;0;0]
      mask Display: e = 0.06;c1 = [120 230 180]/255;c2 = ([120 230 180]+0)/(256+128);c3 = ([120 230 180]+128)/(256+128);patch([0 1 1 0],[0 0 1 1],c1);patch([0 1 1 1-e 1-e 0+e],[0 0 1 1-e 0+e 0+e],c2);patch([0 0 1 1-e 0+e 0+e],[0 1 1 1-e 1-e 0+e],c3);plot([0 1 1 0 0],[0 0 1 1 0]);
  wires:
  tansig/1 -> "a{2}"/1
  netsum/1 -> tansig/1
  "b{2}"/1 -> netsum/2
  "LW{2,1}"/1("lz{2,1}") -> netsum/1
  Delays 1/1("pd{2,1}") -> "LW{2,1}"/1("ad{2,1}")
  "a{1} "/1 -> Delays 1/1("p{2}")

== system AcasXuClosedLoop_m_1/networks/AcasXu_5_1/Layer 3 ==
  "a{2} " : Inport  PortDimensions=50
      mask Display: e = 0.06;c1 = [120 230 180]/255;c2 = ([120 230 180]+0)/(256+128);c3 = ([120 230 180]+128)/(256+128);patch([0 1 1 0],[0 0 1 1],c1);patch([0 1 1 1-e 1-e 0+e],[0 0 1 1-e 0+e 0+e],c2);patch([0 0 1 1-e 0+e 0+e],[0 1 1 1-e 1-e 0+e],c3);plot([0 1 1 0 0],[0 0 1 1 0]);
  Delays 1 : Subsystem
      mask Display: e = 0.06;c1 = [120 150 230]/255;c2 = ([120 150 230]+0)/383;c3 = ([120 150 230]+128)/383;patch([0 1 1 0],[0 0 1 1],c1);patch([0 1 1 1-e 1-e 0+e],[0 0 1 1-e 0+e 0+e],c2);patch([0 0 1 1-e 0+e 0+e],[0 1 1 1-e 1-e 0+e],c3);plot([0 1 1 0 0],[0 0 1 1 0]);disp('0');
  "LW{3,2}" : Subsystem
      mask Display: e = 0.06;c1 = [120 150 230]/255;c2 = ([120 150 230]+0)/383;c3 = ([120 150 230]+128)/383;patch([0 1 1 0],[0 0 1 1],c1);patch([0 1 1 1-e 1-e 0+e],[0 0 1 1-e 0+e 0+e],c2);patch([0 0 1 1-e 0+e 0+e],[0 1 1 1-e 1-e 0+e],c3);plot([0 1 1 0 0],[0 0 1 1 0]);disp('W');
  "b{3}" : Constant  Value=[0.272230000000000027515767442309879697859287261962890625;-1.0544800000000000839150970932678319513797760009765625;1.5729699999999999793232063893810845911502838134765625;1.4368700000000000915889586394769139587879180908203125;-0.422177999999999997715605104531277902424335479736328125;-0.98838400000000004030908939967048354446887969970703125;-0.021854800000000000614885919958396698348224163055419921875;-0.293798999999999976839859527899534441530704498291015625;1.0949400000000000243716158365714363753795623779296875;-0.0307898999999999985199838903326963190920650959014892578125;-0.06296770000000000144790845979514415375888347625732421875;-0.84011599999999997390176531553152017295360565185546875;0.503924000000000038568259697058238089084625244140625;0.2310029999999999861248767274446436204016208648681640625;-0.0287351999999999989376942011176652158610522747039794921875;1.1389400000000000634514663033769465982913970947265625;0.73577899999999996083488440490327775478363037109375;0.110875000000000001332267629550187848508358001708984375;-1.0117599999999999926814098216709680855274200439453125;-0.1491240000000000065494276668687234632670879364013671875;-1.0125100000000000211031192520749755203723907470703125;-1.1087100000000000843414227347238920629024505615234375;1.4243699999999999139532746994518674910068511962890625;0.298072999999999976861175809972337447106838226318359375;0.34876600000000002044231450781808234751224517822265625;0.277681000000000011151968237754772417247295379638671875;-1.259819999999999939888084554695524275302886962890625;-0.26194499999999998340882712000166065990924835205078125;0.14417299999999999560174046564497984945774078369140625;-0.29806100000000002037126023424207232892513275146484375;-1.0689100000000000267874611381557770073413848876953125;-0.0578330999999999983973708594930940307676792144775390625;0.600875999999999965694996717502363026142120361328125;0.61764699999999994606270092845079489052295684814453125;0.65339300000000000157029944602982141077518463134765625;-2.78967000000000009407585821463726460933685302734375;0.57990299999999994629007460389402695000171661376953125;0.480266000000000026215474235868896357715129852294921875;0.343100000000000016076029396572266705334186553955078125;-0.01002399999999999992417176741810180828906595706939697265625;-0.26819300000000001471534005759167484939098358154296875;-0.0729852000000000000756728013584506697952747344970703125;-0.0917779999999999984705567612763843499124050140380859375;0.446454999999999990745180866724695079028606414794921875;0.565514999999999989910293152206577360630035400390625;-0.54441200000000000702726765666739083826541900634765625;0.2388879999999999892423829805920831859111785888671875;0.0464861000000000024190427438952610827982425689697265625;0.55525100000000005007194658901426009833812713623046875;0.09514330000000000009396927680427324958145618438720703125]
      mask Display: e = 0.06;c1 = [120 150 230]/255;c2 = ([120 150 230]+0)/383;c3 = ([120 150 230]+128)/383;patch([0 1 1 0],[0 0 1 1],c1);patch([0 1 1 1-e 1-e 0+e],[0 0 1 1-e 0+e 0+e],c2);patch([0 0 1 1-e 0+e 0+e],[0 1 1 1-e 1-e 0+e],c3);plot([0 1 1 0 0],[0 0 1 1 0]);disp('b');
  netsum : Sum  Inputs=2  SaturateOnIntegerOverflow=on  InputSameDT=on  OutDataTypeStr=Inherit: Same as first input
      mask Display: e = 0.06;c1 = [120 150 230]/255;c2 = ([120 150 230]+0)/383;c3 = ([120 150 230]+128)/383;patch([0 1 1 0],[0 0 1 1],c1);patch([0 1 1 1-e 1-e 0+e],[0 0 1 1-e 0+e 0+e],c2);patch([0 0 1 1-e 0+e 0+e],[0 1 1 1-e 1-e 0+e],c3);plot([0 1 1 0 0],[0 0 1 1 0]);disp('+');
  tansig : neural/Transfer Functions/tansig
      settings: SourceProductName=Deep Learning Toolbox
  "a{3}" : Outport  InitialOutput=[0;0;0;0;0;0;0;0;0;0;0;0;0;0;0;0;0;0;0;0;0;0;0;0;0;0;0;0;0;0;0;0;0;0;0;0;0;0;0;0;0;0;0;0;0;0;0;0;0;0]
      mask Display: e = 0.06;c1 = [120 230 180]/255;c2 = ([120 230 180]+0)/(256+128);c3 = ([120 230 180]+128)/(256+128);patch([0 1 1 0],[0 0 1 1],c1);patch([0 1 1 1-e 1-e 0+e],[0 0 1 1-e 0+e 0+e],c2);patch([0 0 1 1-e 0+e 0+e],[0 1 1 1-e 1-e 0+e],c3);plot([0 1 1 0 0],[0 0 1 1 0]);
  wires:
  tansig/1 -> "a{3}"/1
  netsum/1 -> tansig/1
  "b{3}"/1 -> netsum/2
  "LW{3,2}"/1("lz{3,2}") -> netsum/1
  Delays 1/1("pd{3,2}") -> "LW{3,2}"/1("ad{3,2}")
  "a{2} "/1 -> Delays 1/1("p{3}")

== system AcasXuClosedLoop_m_1/networks/AcasXu_5_1/Layer 4 ==
  "a{3} " : Inport  PortDimensions=50
      mask Display: e = 0.06;c1 = [120 230 180]/255;c2 = ([120 230 180]+0)/(256+128);c3 = ([120 230 180]+128)/(256+128);patch([0 1 1 0],[0 0 1 1],c1);patch([0 1 1 1-e 1-e 0+e],[0 0 1 1-e 0+e 0+e],c2);patch([0 0 1 1-e 0+e 0+e],[0 1 1 1-e 1-e 0+e],c3);plot([0 1 1 0 0],[0 0 1 1 0]);
  Delays 1 : Subsystem
      mask Display: e = 0.06;c1 = [120 150 230]/255;c2 = ([120 150 230]+0)/383;c3 = ([120 150 230]+128)/383;patch([0 1 1 0],[0 0 1 1],c1);patch([0 1 1 1-e 1-e 0+e],[0 0 1 1-e 0+e 0+e],c2);patch([0 0 1 1-e 0+e 0+e],[0 1 1 1-e 1-e 0+e],c3);plot([0 1 1 0 0],[0 0 1 1 0]);disp('0');
  "LW{4,3}" : Subsystem
      mask Display: e = 0.06;c1 = [120 150 230]/255;c2 = ([120 150 230]+0)/383;c3 = ([120 150 230]+128)/383;patch([0 1 1 0],[0 0 1 1],c1);patch([0 1 1 1-e 1-e 0+e],[0 0 1 1-e 0+e 0+e],c2);patch([0 0 1 1-e 0+e 0+e],[0 1 1 1-e 1-e 0+e],c3);plot([0 1 1 0 0],[0 0 1 1 0]);disp('W');
  "b{4}" : Constant  Value=[-0.56321100000000001717381792332162149250507354736328125;-0.08371520000000000349960060930243344046175479888916015625;-1.1247599999999999820232687852694652974605560302734375;-2.294610000000000038511416278197430074214935302734375;0.94715000000000004742872761198668740689754486083984375;0.6754759999999999653397253496223129332065582275390625;-0.0302282000000000002082334304986943607218563556671142578125;-0.0271720000000000017070789226636406965553760528564453125;0.0749916999999999944748196867294609546661376953125;0.269618999999999997552180275306454859673976898193359375;-1.1817299999999999471356204594485461711883544921875;-0.4554139999999999854907173357787542045116424560546875;0.446923000000000014697576489197672344744205474853515625;-0.057709799999999998598720907239112420938909053802490234375;1.61118000000000005655920176650397479534149169921875;-2.418950000000000155608859131461940705776214599609375;-1.77967999999999992866150932968594133853912353515625;1.2901100000000000900257646208046935498714447021484375;0.360455000000000025384139235029579140245914459228515625;-0.78738200000000002631850293255411088466644287109375;0.1540680000000000104964925640160799957811832427978515625;1.3485199999999999409538986583356745541095733642578125;0.429234999999999977671194528738851658999919891357421875;-0.9072050000000000391509047403815202414989471435546875;-0.0237161000000000003751221555603478918783366680145263671875;0.345032999999999978602005512584582902491092681884765625;-0.185626000000000013212542171459062956273555755615234375;-1.07753999999999994230392985627986490726470947265625;0.958077999999999985192289386759512126445770263671875;-0.1085939999999999960866858828012482263147830963134765625;0.70110499999999997822186514895292930305004119873046875;-0.04197879999999999667270600411939085461199283599853515625;0.90369500000000002604139126560767181217670440673828125;0.1236130000000000006554756737386924214661121368408203125;-2.5700599999999997891109160264022648334503173828125;0.1852290000000000047553072590744704939424991607666015625;0.74212599999999995237232042200048454105854034423828125;0.53999699999999994926014323937124572694301605224609375;-0.354986999999999996990851514055975712835788726806640625;1.3218799999999999439381781485280953347682952880859375;-1.9547000000000001040945107888546772301197052001953125;0.74946100000000004381917051432537846267223358154296875;-0.34008300000000002416555844320100732147693634033203125;-0.01237429999999999953586016232520705671049654483795166015625;-2.613170000000000214868123293854296207427978515625;-0.268365000000000020197177263980847783386707305908203125;-0.743109000000000019525714378687553107738494873046875;-2.42053999999999991388222042587585747241973876953125;-0.85676300000000005230305077930097468197345733642578125;-0.75692999999999999172217712839483283460140228271484375]
      mask Display: e = 0.06;c1 = [120 150 230]/255;c2 = ([120 150 230]+0)/383;c3 = ([120 150 230]+128)/383;patch([0 1 1 0],[0 0 1 1],c1);patch([0 1 1 1-e 1-e 0+e],[0 0 1 1-e 0+e 0+e],c2);patch([0 0 1 1-e 0+e 0+e],[0 1 1 1-e 1-e 0+e],c3);plot([0 1 1 0 0],[0 0 1 1 0]);disp('b');
  netsum : Sum  Inputs=2  SaturateOnIntegerOverflow=on  InputSameDT=on  OutDataTypeStr=Inherit: Same as first input
      mask Display: e = 0.06;c1 = [120 150 230]/255;c2 = ([120 150 230]+0)/383;c3 = ([120 150 230]+128)/383;patch([0 1 1 0],[0 0 1 1],c1);patch([0 1 1 1-e 1-e 0+e],[0 0 1 1-e 0+e 0+e],c2);patch([0 0 1 1-e 0+e 0+e],[0 1 1 1-e 1-e 0+e],c3);plot([0 1 1 0 0],[0 0 1 1 0]);disp('+');
  tansig : neural/Transfer Functions/tansig
      settings: SourceProductName=Deep Learning Toolbox
  "a{4}" : Outport  InitialOutput=[0;0;0;0;0;0;0;0;0;0;0;0;0;0;0;0;0;0;0;0;0;0;0;0;0;0;0;0;0;0;0;0;0;0;0;0;0;0;0;0;0;0;0;0;0;0;0;0;0;0]
      mask Display: e = 0.06;c1 = [120 230 180]/255;c2 = ([120 230 180]+0)/(256+128);c3 = ([120 230 180]+128)/(256+128);patch([0 1 1 0],[0 0 1 1],c1);patch([0 1 1 1-e 1-e 0+e],[0 0 1 1-e 0+e 0+e],c2);patch([0 0 1 1-e 0+e 0+e],[0 1 1 1-e 1-e 0+e],c3);plot([0 1 1 0 0],[0 0 1 1 0]);
  wires:
  tansig/1 -> "a{4}"/1
  netsum/1 -> tansig/1
  "b{4}"/1 -> netsum/2
  "LW{4,3}"/1("lz{4,3}") -> netsum/1
  Delays 1/1("pd{4,3}") -> "LW{4,3}"/1("ad{4,3}")
  "a{3} "/1 -> Delays 1/1("p{4}")
